simulink model "Assignment_1_3_PID_Tuning"  (R2023b)
settings: Solver=ode45  StartTime=0.0  StopTime=10  RelTol=1e-3
libraries: simulink x8
settings Model: Creator=User  LastModifiedBy=User

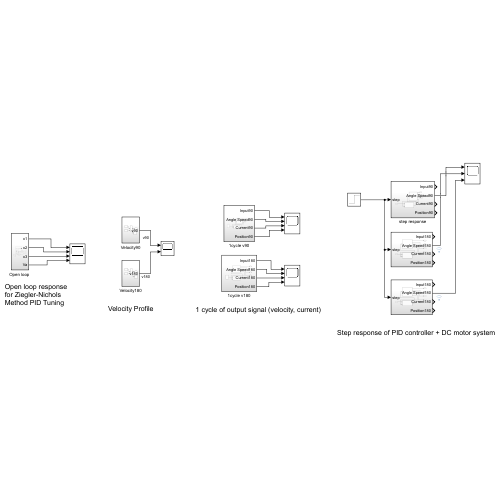
[thumbnail: Simulink's stored preview of the top-level diagram]
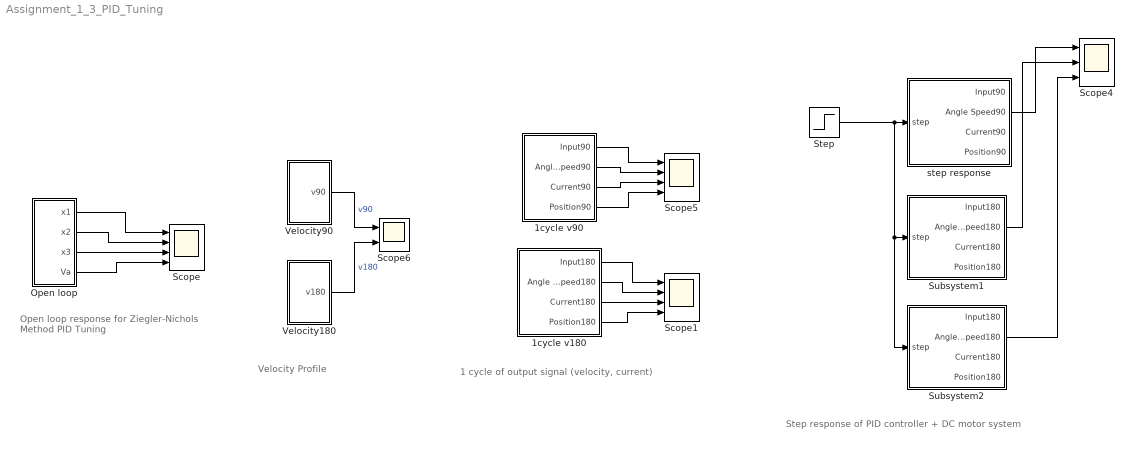
== system Assignment_1_3_PID_Tuning ==
  note: Step response of PID controller + DC motor system
  note: 1 cycle of output signal (velocity, current)
  note: Velocity Profile
  note: Open loop response for Ziegler-Nichols Method PID Tuning
  1cycle v180 : Subsystem
  1cycle v90 : Subsystem
  "Open loop " : Subsystem
  Scope : Scope  NumInputPorts=4
  Scope1 : Scope  NumInputPorts=4
  Scope4 : Scope  NumInputPorts=3
  Scope5 : Scope  NumInputPorts=4
  Scope6 : Scope  NumInputPorts=2
  Step : Step  Time=0  SampleTime=16
  Subsystem1 : Subsystem
  Subsystem2 : Subsystem
  Velocity180 : Subsystem
  Velocity90 : Subsystem
  step response : Subsystem
  wires:
  Velocity180/1(v180) -> Scope6/2  "v180"
  Velocity90/1(v90) -> Scope6/1  "v90"
  1cycle v90/4(Position90) -> Scope5/4
  1cycle v90/2(Angle Speed90) -> Scope5/2
  1cycle v90/3(Current90) -> Scope5/3
  1cycle v90/1(Input90) -> Scope5/1
  step response/2(Angle Speed90) -> Scope4/1
  Step/1 -> Subsystem2/1(step), Subsystem1/1(step), step response/1(step)
  "Open loop "/2(x2) -> Scope/2
  "Open loop "/3(x3) -> Scope/3
  "Open loop "/4(Va) -> Scope/4
  "Open loop "/1(x1) -> Scope/1
  1cycle v180/3(Current180) -> Scope1/3
  1cycle v180/1(Input180) -> Scope1/1
  1cycle v180/2(Angle Speed180) -> Scope1/2
  1cycle v180/4(Position180) -> Scope1/4
  Subsystem1/2(Angle Speed180) -> Scope4/2
  Subsystem2/2(Angle Speed180) -> Scope4/3

== system Assignment_1_3_PID_Tuning/1cycle v180 ==
  DC motor : Subsystem
  PID : Subsystem
  Velocity 180 : Subsystem
  Input180 : Outport
  Angle Speed180 : Outport  Port=2
  Current180 : Outport  Port=3
  Position180 : Outport  Port=4
  wires:
  DC motor/5(w,x180) -> PID/2(In 2)  "feedback loop"
  DC motor/2(Angle Speed180) -> Angle Speed180/1
  DC motor/3(Current180) -> Current180/1
  Velocity 180/1(v180) -> PID/1(va)
  DC motor/4(Position180) -> Position180/1
  DC motor/1(Input180) -> Input180/1
  PID/1(w,x180) -> DC motor/1(In 2)

== system Assignment_1_3_PID_Tuning/1cycle v90 ==
  Subsystem3 : Subsystem
  Subsystem4 : Subsystem
  Velocity 90 : Subsystem
  Input90 : Outport
  Angle Speed90 : Outport  Port=2
  Current90 : Outport  Port=3
  Position90 : Outport  Port=4
  wires:
  Subsystem4/1(w,x90) -> Subsystem3/1(In 1)
  Velocity 90/1(v90) -> Subsystem4/1(v90)
  Subsystem3/4(Position90) -> Position90/1
  Subsystem3/5(w,x90) -> Subsystem4/2(In 1)
  Subsystem3/3(Current90) -> Current90/1
  Subsystem3/1(Input90) -> Input90/1
  Subsystem3/2(Angle Speed90) -> Angle Speed90/1

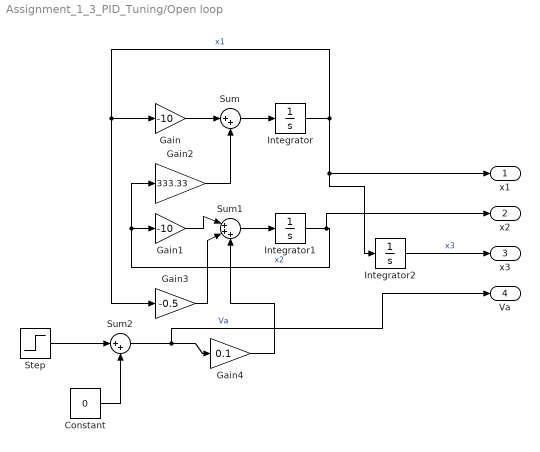
== system Assignment_1_3_PID_Tuning/Open loop  ==
  Constant : Constant  Value=0
  Gain : Gain  Gain=-10
  Gain1 : Gain  Gain=-10
  Gain2 : Gain  Gain=333.33
  Gain3 : Gain  Gain=-0.5
  Gain4 : Gain  Gain=0.1
  Integrator : Integrator
  Integrator1 : Integrator
  Integrator2 : Integrator
  Step : Step  Time=0  SampleTime=32
  Sum : Sum  Inputs=|++
  Sum1 : Sum  Inputs=|+++
  Sum2 : Sum  Inputs=|++
  x1 : Outport
  x2 : Outport  Port=2
  x3 : Outport  Port=3
  Va : Outport  Port=4
  wires:
  Integrator1/1 -> x2/1, Gain2/1, Gain1/1  "x2"
  Integrator/1 -> Gain/1, Gain3/1, x1/1, Integrator2/1  "x1"
  Sum/1 -> Integrator/1
  Sum2/1 -> Va/1, Gain4/1  "Va"
  Gain1/1 -> Sum1/1
  Constant/1 -> Sum2/2
  Gain4/1 -> Sum1/3
  Gain2/1 -> Sum/2
  Gain/1 -> Sum/1
  Sum1/1 -> Integrator1/1
  Gain3/1 -> Sum1/2
  Step/1 -> Sum2/1
  Integrator2/1 -> x3/1  "x3"

== system Assignment_1_3_PID_Tuning/Subsystem1 ==
  step : Inport
  DC motor : Subsystem
  PID : Subsystem
  Input180 : Outport
  Angle Speed180 : Outport  Port=2
  Current180 : Outport  Port=3
  Position180 : Outport  Port=4
  wires:
  DC motor/3(Current180) -> Current180/1
  PID/1(w,x180) -> DC motor/1(In 2)
  DC motor/2(Angle Speed180) -> Angle Speed180/1
  DC motor/1(Input180) -> Input180/1
  DC motor/5(w,x180) -> PID/2(In 2)  "feedback loop"
  DC motor/4(Position180) -> Position180/1
  step/1 -> PID/1(v180)

== system Assignment_1_3_PID_Tuning/Subsystem2 ==
  step : Inport
  DC motor : Subsystem
  PID : Subsystem
  Input180 : Outport
  Angle Speed180 : Outport  Port=2
  Current180 : Outport  Port=3
  Position180 : Outport  Port=4
  wires:
  DC motor/3(Current180) -> Current180/1
  PID/1(w,x180) -> DC motor/1(In 2)
  DC motor/2(Angle Speed180) -> Angle Speed180/1
  DC motor/1(Input180) -> Input180/1
  DC motor/5(w,x180) -> PID/2(In 2)  "feedback loop"
  DC motor/4(Position180) -> Position180/1
  step/1 -> PID/1(v180)

== system Assignment_1_3_PID_Tuning/Velocity180 ==
  Scope7 : Scope
  Sum1 : Sum  Inputs=|++
  vpick+drop : simulink/Sources/Repeating Sequence  rep_seq_t=[0 0.25 1 1.25 1.5 1.75 2.5 2.75 3 16]  rep_seq_y=[0 pi/2 pi/2 0 0 -pi/2 -pi/2 0 0 0]
  w180 : simulink/Sources/Repeating Sequence  rep_seq_t="[0 3 3.25 5  5.25 5.5 5.75 7.5 7.75 8 16]"  rep_seq_y=[0 0 pi/2 pi/2 0 0 -pi/2 -pi/2 0 0 0]
  v180 : Outport
  wires:
  w180/1 -> Sum1/1
  Sum1/1 -> v180/1, Scope7/1
  vpick+drop/1 -> Sum1/2

== system Assignment_1_3_PID_Tuning/Velocity90 ==
  Scope4 : Scope
  Sum : Sum  Inputs=|++
  vpick+drop : simulink/Sources/Repeating Sequence  rep_seq_t=[0 0.25 1 1.25 1.5 1.75 2.5 2.75 3 16]  rep_seq_y=[0 pi/2 pi/2 0 0 -pi/2 -pi/2 0 0 0]
  w90 : simulink/Sources/Repeating Sequence  rep_seq_t=[0 3 3.25 4 4.25 4.5 4.75 5.5 5.75 6 16]  rep_seq_y=[0 0 pi/2 pi/2 0 0 -pi/2 -pi/2 0 0 0]
  v90 : Outport
  wires:
  vpick+drop/1 -> Sum/1
  w90/1 -> Sum/2
  Sum/1 -> v90/1, Scope4/1

== system Assignment_1_3_PID_Tuning/step response ==
  step : Inport
  Subsystem1 : Subsystem
  Subsystem2 : Subsystem
  Input90 : Outport
  Angle Speed90 : Outport  Port=2
  Current90 : Outport  Port=3
  Position90 : Outport  Port=4
  wires:
  Subsystem1/5(w,x90) -> Subsystem2/2(In 1)
  Subsystem1/4(Position90) -> Position90/1
  Subsystem2/1(w,x90) -> Subsystem1/1(In 1)
  Subsystem1/3(Current90) -> Current90/1
  Subsystem1/1(Input90) -> Input90/1
  step/1 -> Subsystem2/1(v90)
  Subsystem1/2(Angle Speed90) -> Angle Speed90/1

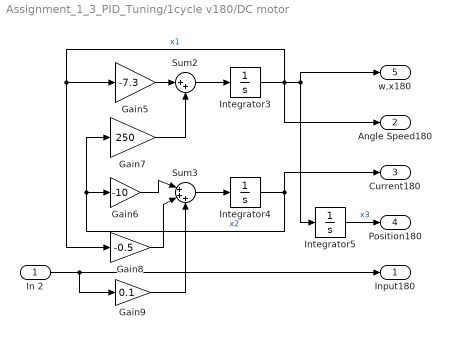
== system Assignment_1_3_PID_Tuning/1cycle v180/DC motor ==
  In 2 : Inport
  Gain5 : Gain  Gain=-7.3
  Gain6 : Gain  Gain=-10
  Gain7 : Gain  Gain=250
  Gain8 : Gain  Gain=-0.5
  Gain9 : Gain  Gain=0.1
  Integrator3 : Integrator
  Integrator4 : Integrator
  Integrator5 : Integrator
  Sum2 : Sum  Inputs=|++
  Sum3 : Sum  Inputs=|+++
  Input180 : Outport
  Angle Speed180 : Outport  Port=2
  Current180 : Outport  Port=3
  Position180 : Outport  Port=4
  w,x180 : Outport  Port=5
  wires:
  Integrator4/1 -> Current180/1, Gain7/1, Gain6/1  "x2"
  Gain7/1 -> Sum2/2
  Gain6/1 -> Sum3/1
  Sum2/1 -> Integrator3/1
  Gain9/1 -> Sum3/3
  Gain8/1 -> Sum3/2
  Sum3/1 -> Integrator4/1
  Integrator3/1 -> Gain8/1, Gain5/1, Angle Speed180/1, Integrator5/1, w,x180/1  "x1"
  Gain5/1 -> Sum2/1
  Integrator5/1 -> Position180/1  "x3"
  In 2/1 -> Gain9/1, Input180/1

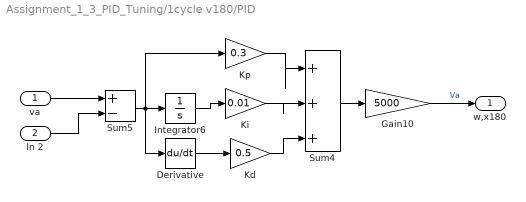
== system Assignment_1_3_PID_Tuning/1cycle v180/PID ==
  va : Inport
  In 2 : Inport  Port=2
  Derivative : Derivative
  Gain10 : Gain  Gain=5000
  Integrator6 : Integrator
  Kd : Gain  Gain=0.5
  Ki : Gain  Gain=0.01
  Kp : Gain  Gain=0.3
  Sum4 : Sum  Inputs=|+++
  Sum5 : Sum  Inputs=+-
  w,x180 : Outport
  wires:
  Kp/1 -> Sum4/1
  Derivative/1 -> Kd/1
  Sum5/1 -> Integrator6/1, Kp/1, Derivative/1
  Ki/1 -> Sum4/2
  va/1 -> Sum5/1
  Sum4/1 -> Gain10/1
  Gain10/1 -> w,x180/1  "Va"
  Kd/1 -> Sum4/3
  Integrator6/1 -> Ki/1
  In 2/1 -> Sum5/2

== system Assignment_1_3_PID_Tuning/1cycle v180/Velocity 180 ==
  Scope5 : Scope
  Scope6 : Scope
  Scope7 : Scope
  Sum1 : Sum  Inputs=|++
  vpick+drop : simulink/Sources/Repeating Sequence  rep_seq_t=[0 0.25 1 1.25 1.5 1.75 2.5 2.75 3 16]  rep_seq_y=[0 pi/2 pi/2 0 0 -pi/2 -pi/2 0 0 0]
  w180 : simulink/Sources/Repeating Sequence  rep_seq_t="[0 3 3.25 5  5.25 5.5 5.75 7.5 7.75 8 16]"  rep_seq_y=[0 0 pi/2 pi/2 0 0 -pi/2 -pi/2 0 0 0]
  v180 : Outport
  wires:
  w180/1 -> Sum1/1, Scope5/1
  Sum1/1 -> v180/1, Scope7/1
  vpick+drop/1 -> Scope6/1, Sum1/2

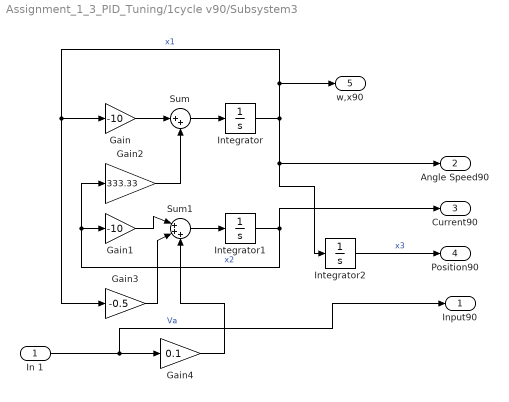
== system Assignment_1_3_PID_Tuning/1cycle v90/Subsystem3 ==
  In 1 : Inport
  Gain : Gain  Gain=-10
  Gain1 : Gain  Gain=-10
  Gain2 : Gain  Gain=333.33
  Gain3 : Gain  Gain=-0.5
  Gain4 : Gain  Gain=0.1
  Integrator : Integrator
  Integrator1 : Integrator
  Integrator2 : Integrator
  Sum : Sum  Inputs=|++
  Sum1 : Sum  Inputs=|+++
  Input90 : Outport
  Angle Speed90 : Outport  Port=2
  Current90 : Outport  Port=3
  Position90 : Outport  Port=4
  w,x90 : Outport  Port=5
  wires:
  Integrator/1 -> w,x90/1, Gain/1, Gain3/1, Angle Speed90/1, Integrator2/1  "x1"
  Sum1/1 -> Integrator1/1
  Gain/1 -> Sum/1
  Sum/1 -> Integrator/1
  Gain4/1 -> Sum1/3
  Integrator1/1 -> Current90/1, Gain2/1, Gain1/1  "x2"
  Gain3/1 -> Sum1/2
  Integrator2/1 -> Position90/1  "x3"
  Gain1/1 -> Sum1/1
  Gain2/1 -> Sum/2
  In 1/1 -> Input90/1, Gain4/1  "Va"

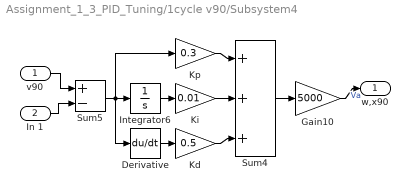
== system Assignment_1_3_PID_Tuning/1cycle v90/Subsystem4 ==
  v90 : Inport
  In 1 : Inport  Port=2
  Derivative : Derivative
  Gain10 : Gain  Gain=5000
  Integrator6 : Integrator
  Kd : Gain  Gain=0.5
  Ki : Gain  Gain=0.01
  Kp : Gain  Gain=0.3
  Sum4 : Sum  Inputs=|+++
  Sum5 : Sum  Inputs=+-
  w,x90 : Outport
  wires:
  Kp/1 -> Sum4/1
  Derivative/1 -> Kd/1
  Sum5/1 -> Kp/1, Integrator6/1, Derivative/1
  Ki/1 -> Sum4/2
  Sum4/1 -> Gain10/1
  Gain10/1 -> w,x90/1  "Va"
  Kd/1 -> Sum4/3
  Integrator6/1 -> Ki/1
  In 1/1 -> Sum5/2
  v90/1 -> Sum5/1

== system Assignment_1_3_PID_Tuning/1cycle v90/Velocity 90 ==
  Scope2 : Scope
  Scope3 : Scope
  Scope4 : Scope
  Sum : Sum  Inputs=|++
  vpick+drop : simulink/Sources/Repeating Sequence  rep_seq_t=[0 0.25 1 1.25 1.5 1.75 2.5 2.75 3 16]  rep_seq_y=[0 pi/2 pi/2 0 0 -pi/2 -pi/2 0 0 0]
  w90 : simulink/Sources/Repeating Sequence  rep_seq_t=[0 3 3.25 4 4.25 4.5 4.75 5.5 5.75 6 16]  rep_seq_y=[0 0 pi/2 pi/2 0 0 -pi/2 -pi/2 0 0 0]
  v90 : Outport
  wires:
  vpick+drop/1 -> Sum/1, Scope2/1
  w90/1 -> Sum/2, Scope3/1
  Sum/1 -> v90/1, Scope4/1

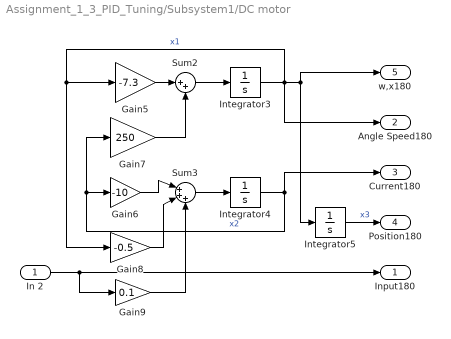
== system Assignment_1_3_PID_Tuning/Subsystem1/DC motor ==
  In 2 : Inport
  Gain5 : Gain  Gain=-7.3
  Gain6 : Gain  Gain=-10
  Gain7 : Gain  Gain=250
  Gain8 : Gain  Gain=-0.5
  Gain9 : Gain  Gain=0.1
  Integrator3 : Integrator
  Integrator4 : Integrator
  Integrator5 : Integrator
  Sum2 : Sum  Inputs=|++
  Sum3 : Sum  Inputs=|+++
  Input180 : Outport
  Angle Speed180 : Outport  Port=2
  Current180 : Outport  Port=3
  Position180 : Outport  Port=4
  w,x180 : Outport  Port=5
  wires:
  Integrator4/1 -> Current180/1, Gain7/1, Gain6/1  "x2"
  Gain7/1 -> Sum2/2
  Gain6/1 -> Sum3/1
  Sum2/1 -> Integrator3/1
  Gain9/1 -> Sum3/3
  Gain8/1 -> Sum3/2
  Sum3/1 -> Integrator4/1
  Integrator3/1 -> Gain8/1, Gain5/1, Angle Speed180/1, Integrator5/1, w,x180/1  "x1"
  Gain5/1 -> Sum2/1
  Integrator5/1 -> Position180/1  "x3"
  In 2/1 -> Gain9/1, Input180/1

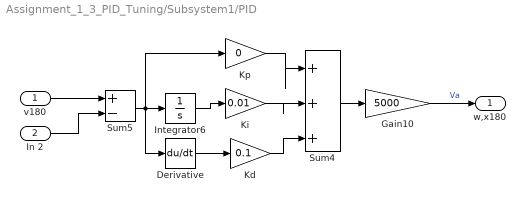
== system Assignment_1_3_PID_Tuning/Subsystem1/PID ==
  v180 : Inport
  In 2 : Inport  Port=2
  Derivative : Derivative
  Gain10 : Gain  Gain=5000
  Integrator6 : Integrator
  Kd : Gain  Gain=0.1
  Ki : Gain  Gain=0.01
  Kp : Gain  Gain=0
  Sum4 : Sum  Inputs=|+++
  Sum5 : Sum  Inputs=+-
  w,x180 : Outport
  wires:
  Kp/1 -> Sum4/1
  Derivative/1 -> Kd/1
  Sum5/1 -> Integrator6/1, Kp/1, Derivative/1
  Ki/1 -> Sum4/2
  v180/1 -> Sum5/1
  Sum4/1 -> Gain10/1
  Gain10/1 -> w,x180/1  "Va"
  Kd/1 -> Sum4/3
  Integrator6/1 -> Ki/1
  In 2/1 -> Sum5/2

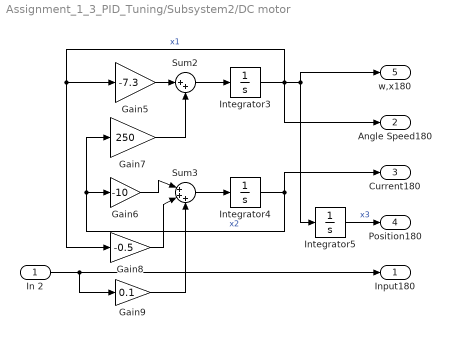
== system Assignment_1_3_PID_Tuning/Subsystem2/DC motor ==
  In 2 : Inport
  Gain5 : Gain  Gain=-7.3
  Gain6 : Gain  Gain=-10
  Gain7 : Gain  Gain=250
  Gain8 : Gain  Gain=-0.5
  Gain9 : Gain  Gain=0.1
  Integrator3 : Integrator
  Integrator4 : Integrator
  Integrator5 : Integrator
  Sum2 : Sum  Inputs=|++
  Sum3 : Sum  Inputs=|+++
  Input180 : Outport
  Angle Speed180 : Outport  Port=2
  Current180 : Outport  Port=3
  Position180 : Outport  Port=4
  w,x180 : Outport  Port=5
  wires:
  Integrator4/1 -> Current180/1, Gain7/1, Gain6/1  "x2"
  Gain7/1 -> Sum2/2
  Gain6/1 -> Sum3/1
  Sum2/1 -> Integrator3/1
  Gain9/1 -> Sum3/3
  Gain8/1 -> Sum3/2
  Sum3/1 -> Integrator4/1
  Integrator3/1 -> Gain8/1, Gain5/1, Angle Speed180/1, Integrator5/1, w,x180/1  "x1"
  Gain5/1 -> Sum2/1
  Integrator5/1 -> Position180/1  "x3"
  In 2/1 -> Gain9/1, Input180/1

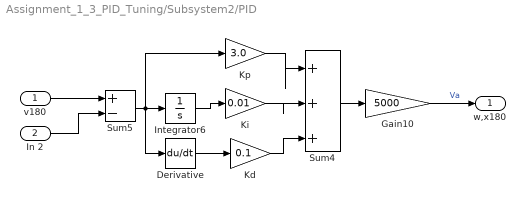
== system Assignment_1_3_PID_Tuning/Subsystem2/PID ==
  v180 : Inport
  In 2 : Inport  Port=2
  Derivative : Derivative
  Gain10 : Gain  Gain=5000
  Integrator6 : Integrator
  Kd : Gain  Gain=0.1
  Ki : Gain  Gain=0.01
  Kp : Gain  Gain=3.0
  Sum4 : Sum  Inputs=|+++
  Sum5 : Sum  Inputs=+-
  w,x180 : Outport
  wires:
  Kp/1 -> Sum4/1
  Derivative/1 -> Kd/1
  Sum5/1 -> Integrator6/1, Kp/1, Derivative/1
  Ki/1 -> Sum4/2
  v180/1 -> Sum5/1
  Sum4/1 -> Gain10/1
  Gain10/1 -> w,x180/1  "Va"
  Kd/1 -> Sum4/3
  Integrator6/1 -> Ki/1
  In 2/1 -> Sum5/2

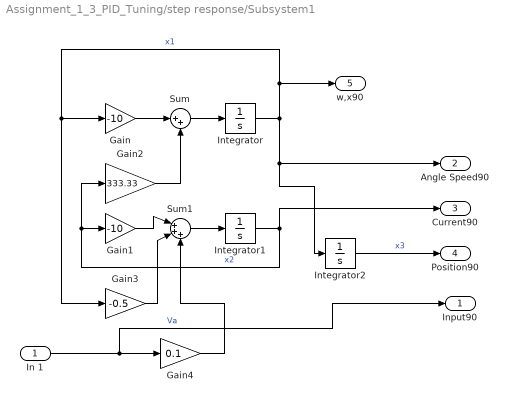
== system Assignment_1_3_PID_Tuning/step response/Subsystem1 ==
  In 1 : Inport
  Gain : Gain  Gain=-10
  Gain1 : Gain  Gain=-10
  Gain2 : Gain  Gain=333.33
  Gain3 : Gain  Gain=-0.5
  Gain4 : Gain  Gain=0.1
  Integrator : Integrator
  Integrator1 : Integrator
  Integrator2 : Integrator
  Sum : Sum  Inputs=|++
  Sum1 : Sum  Inputs=|+++
  Input90 : Outport
  Angle Speed90 : Outport  Port=2
  Current90 : Outport  Port=3
  Position90 : Outport  Port=4
  w,x90 : Outport  Port=5
  wires:
  Integrator/1 -> w,x90/1, Gain/1, Gain3/1, Angle Speed90/1, Integrator2/1  "x1"
  Sum1/1 -> Integrator1/1
  Gain/1 -> Sum/1
  Sum/1 -> Integrator/1
  Gain4/1 -> Sum1/3
  Integrator1/1 -> Current90/1, Gain2/1, Gain1/1  "x2"
  Gain3/1 -> Sum1/2
  Integrator2/1 -> Position90/1  "x3"
  Gain1/1 -> Sum1/1
  Gain2/1 -> Sum/2
  In 1/1 -> Input90/1, Gain4/1  "Va"

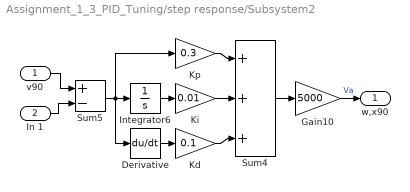
== system Assignment_1_3_PID_Tuning/step response/Subsystem2 ==
  v90 : Inport
  In 1 : Inport  Port=2
  Derivative : Derivative
  Gain10 : Gain  Gain=5000
  Integrator6 : Integrator
  Kd : Gain  Gain=0.1
  Ki : Gain  Gain=0.01
  Kp : Gain  Gain=0.3
  Sum4 : Sum  Inputs=|+++
  Sum5 : Sum  Inputs=+-
  w,x90 : Outport
  wires:
  Kp/1 -> Sum4/1
  Derivative/1 -> Kd/1
  Sum5/1 -> Kp/1, Integrator6/1, Derivative/1
  Ki/1 -> Sum4/2
  Sum4/1 -> Gain10/1
  Gain10/1 -> w,x90/1  "Va"
  Kd/1 -> Sum4/3
  Integrator6/1 -> Ki/1
  In 1/1 -> Sum5/2
  v90/1 -> Sum5/1
